simulink library "powerlib_extras"  (Simulink 6.0)
settings: Solver=ode45  SolverMode=SingleTasking  StartTime=0.0  StopTime=10.0  RelTol=1e-3
undefined symbols (not defined in the file or in its folder): Ac, Bc, Cc, Dc, Delay_discrete, dend, DiscIntNeverNeededParam, extra_sc, j, numd, test_alpha, Ts
libraries: powerlib2 x112, powerlib_extras x70, simulink_extras x25, simulink x12, powerlib_models x8
(part 7 of 9)

== system powerlib_extras/Discrete  Control Blocks/Discrete 12-Pulse HVDC Control /2nd order BP filters ==
  A : Inport  Port=1  LatchInput=off
  B : Inport  Port=2  LatchInput=off
  C : Inport  Port=3  LatchInput=off
  Discrete  2nd-Order FilterA : powerlib_extras/Discrete  Control Blocks/Discrete  2nd-Order Filter  FilterType=Bandpass  Fo=f0  Zeta=BP/2/f0  Ts=pas  Initialize=off  Vac_Init=[0.8 -25 60]  Vdc_Init=-0.4  PlotResponse=off  param1=[1 500 0.1]
  Discrete  2nd-Order FilterB : powerlib_extras/Discrete  Control Blocks/Discrete  2nd-Order Filter  FilterType=Bandpass  Fo=f0  Zeta=BP/2/f0  Ts=pas  Initialize=off  Vac_Init=[0.8 -25 60]  Vdc_Init=-0.4  PlotResponse=off  param1=[1 500 0.1]
  Discrete  2nd-Order FilterC : powerlib_extras/Discrete  Control Blocks/Discrete  2nd-Order Filter  FilterType=Bandpass  Fo=f0  Zeta=BP/2/f0  Ts=pas  Initialize=off  Vac_Init=[0.8 -25 60]  Vdc_Init=-0.4  PlotResponse=off  param1=[1 500 0.1]
  "A " : Outport
  "B " : Outport  Port=2
  "C " : Outport  Port=3
  wires:
  Discrete  2nd-Order FilterC/1 -> "C "/1
  C/1 -> Discrete  2nd-Order FilterC/1
  Discrete  2nd-Order FilterB/1 -> "B "/1
  B/1 -> Discrete  2nd-Order FilterB/1
  Discrete  2nd-Order FilterA/1 -> "A "/1
  A/1 -> Discrete  2nd-Order FilterA/1

== system powerlib_extras/Discrete  Control Blocks/Discrete 12-Pulse HVDC Control /Alpha Control ==
  alpha_max : Inport  Port=1  LatchInput=off
  alpha_min : Inport  Port=2  LatchInput=off
  forced delay : Inport  Port=3  LatchInput=off
  Data Type  Conversion : DataTypeConversion  Orientation=up  OutDataTypeMode=boolean  SaturateOnIntegerOverflow=on  RndMeth=Zero
  Data Type  Conversion1 : DataTypeConversion  OutDataTypeMode=boolean  SaturateOnIntegerOverflow=on  RndMeth=Zero
  Logical Operator : Logic  Operator=OR
  Switch : Switch  Threshold=0.5  SaturateOnIntegerOverflow=on  InputSameDT=on
  Switch1 : Switch  Threshold=0.5  SaturateOnIntegerOverflow=on  InputSameDT=on
  alpha_min_inv (deg)2 : Constant  Value=test_alpha
  fixed alpha (degrees) : Constant  Value=alpha_fix
  max_i : Outport
  min_i : Outport  Port=2
  wires:
  Data Type  Conversion1/1 -> Logical Operator/1
  alpha_min_inv (deg)2/1 -> Data Type  Conversion1/1
  Data Type  Conversion/1 -> Logical Operator/2
  forced delay/1 -> Data Type  Conversion/1
  fixed alpha (degrees)/1 -> Switch1/1, Switch/1
  Switch1/1 -> min_i/1
  Switch/1 -> max_i/1
  alpha_min/1 -> Switch1/3
  alpha_max/1 -> Switch/3
  Logical Operator/1 -> Switch1/2, Switch/2  "alpha i control"

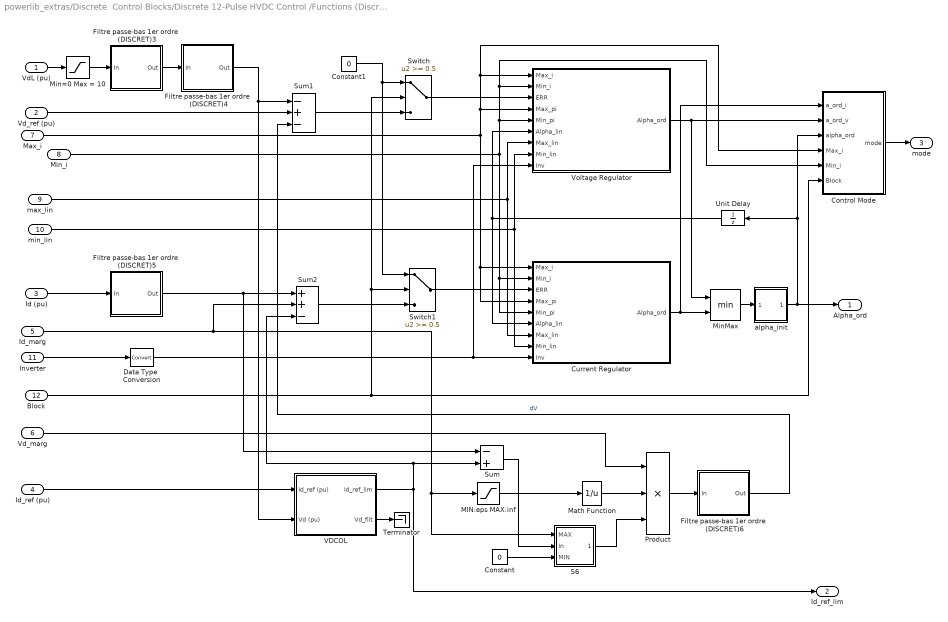
== system powerlib_extras/Discrete  Control Blocks/Discrete 12-Pulse HVDC Control /Functions (Discrete) ==
  VdL (pu) : Inport  Port=1  LatchInput=off
  Vd_ref (pu) : Inport  Port=2  LatchInput=off
  Id (pu) : Inport  Port=3  LatchInput=off
  Id_ref (pu) : Inport  Port=4  LatchInput=off
  Id_marg : Inport  Port=5  LatchInput=off
  Vd_marg : Inport  Port=6  LatchInput=off
  Max_i : Inport  Port=7  LatchInput=off
  Min_i : Inport  Port=8  LatchInput=off
  max_lin : Inport  Port=9  LatchInput=off
  min_lin : Inport  Port=10  LatchInput=off
  Inverter : Inport  Port=11  LatchInput=off
  Block : Inport  Port=12  LatchInput=off
  Constant : Constant  Value=0
  Constant1 : Constant  Value=0
  Control Mode : Subsystem
  Current Regulator : Subsystem  mask(PI Regulator  With  External  Limits (Discrete)){Kp=Kp_I, Ki=Ki_I, IC_i=ICi_I, On_lin=on, pas=pas}
      mask prompts: Kp "Kp (deg/pu):"; Ki "Ki (deg/pu/s):"; IC_i "Integrator Initial Condition (deg):"; On_lin "Linearization  (On)"; pas "Sample time (s):"
      mask help: For the linearization it is important to specifie the mode of operation i.e. rectifier or inverter (negation of rectifier).
      mask Display: disp('PI Regulator\nWith external limits\n(Linearized Kp)\n(Discrete)\n\n')
  Data Type  Conversion : DataTypeConversion  OutDataTypeMode=boolean  SaturateOnIntegerOverflow=on  RndMeth=Zero
  Filtre passe-bas 1er ordre  (DISCRET)3 : Subsystem  mask(First Order Low Pass Filter (Discrete)){T=T1_V, Pas=pas}
      mask prompts: T "Time constant T (s) :"; Pas "Time step (s)"
      mask help: H(s)=1/(1+T.s)
      mask init:
      | X=[0 1 2 3 4];
      | Y=[-2 -2 -3 -4 -4];
      | str=sprintf('\nH=1/(1+T.s)\n T= %g s\n\n\n',T);
      | num=1;
      | den=[T 1];
      | if exist('control/tf/tf')
      |    sys=tf(num,den);
      |    sysd=c2d(sys,Pas,'tustin');
      |    sys=tf(sysd);
      |    [numd,dend]=tfdata(sys,'v');
      | else
      |    [a,b,c,d]=tf2ss(num,den);
      |    nstates = size(a,1);
      |    invexp = inv(eye(nstates) - (Pas/2)*a);
      |    aout = invexp*(eye(nstates) + (Pas/2)*a);
      |    bout = invexp*b;
      |    cout = c*invexp*Pas;
      |    dout = c*invexp*b*(Pas/2) + d;
      |    [numd,dend]=ss2tf(aout,bout,cout,dout,1);
      | end
      mask Display:
      | plot(X,Y);
      | disp(str);
  Filtre passe-bas 1er ordre  (DISCRET)4 : Subsystem  mask(First Order Low Pass Filter (Discrete)){T=T2_V, Pas=pas}
      mask prompts: T "Time constant T (s) :"; Pas "Time step (s)"
      mask help: H(s)=1/(1+T.s)
      mask init: same as powerlib_extras/Discrete  Control Blocks/Discrete 12-Pulse HVDC Control /Functions (Discrete)/Filtre passe-bas 1er ordre  (DISCRET)3
      mask Display:
      | plot(X,Y);
      | disp(str);
  Filtre passe-bas 1er ordre  (DISCRET)5 : Subsystem  mask(First Order Low Pass Filter (Discrete)){T=T1_I, Pas=pas}
      mask prompts: T "Time constant T (s) :"; Pas "Time step (s)"
      mask help: H(s)=1/(1+T.s)
      mask init: same as powerlib_extras/Discrete  Control Blocks/Discrete 12-Pulse HVDC Control /Functions (Discrete)/Filtre passe-bas 1er ordre  (DISCRET)3
      mask Display:
      | plot(X,Y);
      | disp(str);
  Filtre passe-bas 1er ordre  (DISCRET)6 : Subsystem  mask(First Order Low Pass Filter (Discrete)){T=0.2, Pas=pas}
      mask prompts: T "Time constant T (s) :"; Pas "Time step (s)"
      mask help: H(s)=1/(1+T.s)
      mask init: same as powerlib_extras/Discrete  Control Blocks/Discrete 12-Pulse HVDC Control /Functions (Discrete)/Filtre passe-bas 1er ordre  (DISCRET)3
      mask Display:
      | plot(X,Y);
      | disp(str);
  MIN:eps MAX:inf : Saturate  UpperLimit=inf  LowerLimit=eps
  Math Function : Math  Operator=reciprocal  SaturateOnIntegerOverflow=on
  Min=0 Max = 10 : Saturate  UpperLimit=10  LowerLimit=0
  MinMax : MinMax  Inputs=2  SaturateOnIntegerOverflow=on  InputSameDT=on
  Product : Product  Inputs=3  SaturateOnIntegerOverflow=on  InputSameDT=on
  S6 : Subsystem
      mask Type: Limiter with External Limits
      mask Display: disp('      Limiter\n')
  Sum : Sum  Inputs=-+  SaturateOnIntegerOverflow=on  InputSameDT=on
  Sum1 : Sum  Inputs=-+-  SaturateOnIntegerOverflow=on  InputSameDT=on
  Sum2 : Sum  Inputs=++-  SaturateOnIntegerOverflow=on  InputSameDT=on
  Switch : Switch  Threshold=0.5  SaturateOnIntegerOverflow=on  InputSameDT=on
  Switch1 : Switch  Threshold=0.5  SaturateOnIntegerOverflow=on  InputSameDT=on
  Terminator : Terminator
  Unit Delay : UnitDelay  Orientation=left  SampleTime=pas
  VDCOL : Subsystem  mask(Voltage Dependent Current Order Limiter  (Discrete)){Vd_seuil=Vd_seuil, Vd_min=Vd_min, Id_min=Id_min, Id_min_abs=Id_min_abs, Tu=Tup, pas=pas}
      mask prompts: Vd_seuil "Vd seuil (pu):"; Vd_min "Vd min (pu):"; Id_min "Id min (pu):"; Id_min_abs "Id min abs (pu):"; Tu "Up Time constant (s):"; pas "Sample time (s):"
      mask Display: disp('VDCOL\n (Discrete)')
  Voltage Regulator : Subsystem  mask(PI Regulator  With  External  Limits (Discrete)){Kp=Kp_V, Ki=Ki_V, IC_i=ICi_V, On_lin=on, pas=pas}
      mask prompts: Kp "Kp (deg/pu):"; Ki "Ki (deg/pu/s):"; IC_i "Integrator Initial Condition (deg):"; On_lin "Linearization  (On)"; pas "Sample time (s):"
      mask help: For the linearization it is important to specifie the mode of operation i.e. rectifier or inverter (negation of rectifier).
      mask Display: disp('PI Regulator\nWith external limits\n(Linearized Kp)\n(Discrete)\n\n')
  alpha_init : Subsystem
  Alpha_ord : Outport
  Id_ref_lim : Outport  Port=2
  mode : Outport  Port=3
  wires:
  Id_marg/1 -> Sum2/2, S6/1(MAX), MIN:eps MAX:inf/1
  Vd_ref (pu)/1 -> Sum1/2
  Id_ref (pu)/1 -> VDCOL/1(Id_ref (pu))
  Sum/1 -> S6/2(In)
  Constant/1 -> S6/3(MIN)
  VDCOL/2(Vd_filt) -> Terminator/1
  VDCOL/1(Id_ref_lim) -> Id_ref_lim/1, Sum/2, Sum2/3
  MIN:eps MAX:inf/1 -> Math Function/1
  Filtre passe-bas 1er ordre  (DISCRET)4/1(Out) -> VDCOL/2(Vd (pu)), Sum1/1
  Filtre passe-bas 1er ordre  (DISCRET)3/1(Out) -> Filtre passe-bas 1er ordre  (DISCRET)4/1(In)
  Min=0 Max = 10/1 -> Filtre passe-bas 1er ordre  (DISCRET)3/1(In)
  VdL (pu)/1 -> Min=0 Max = 10/1
  Id (pu)/1 -> Filtre passe-bas 1er ordre  (DISCRET)5/1(In)
  Filtre passe-bas 1er ordre  (DISCRET)5/1(Out) -> Sum/1, Sum2/1
  Sum1/1 -> Switch/3
  Sum2/1 -> Switch1/3
  MinMax/1 -> alpha_init/1(In1)
  Unit Delay/1 -> Current Regulator/6(Alpha_lin), Voltage Regulator/6(Alpha_lin)
  S6/1("  ") -> Product/3
  Product/1 -> Filtre passe-bas 1er ordre  (DISCRET)6/1(In)
  Vd_marg/1 -> Product/1
  Math Function/1 -> Product/2
  alpha_init/1(Out1) -> Alpha_ord/1, Unit Delay/1, Control Mode/3(alpha_ord)
  max_lin/1 -> Voltage Regulator/7(Max_lin), Current Regulator/7(Max_lin)
  min_lin/1 -> Voltage Regulator/8(Min_lin), Current Regulator/8(Min_lin)
  Filtre passe-bas 1er ordre  (DISCRET)6/1(Out) -> Sum1/3  "dV"
  Current Regulator/1(Alpha_ord) -> MinMax/2, Control Mode/1("a_ord_i ")
  Voltage Regulator/1(Alpha_ord) -> MinMax/1, Control Mode/2(a_ord_v)
  Max_i/1 -> Current Regulator/4(Max_pi), Current Regulator/1(Max_i), Voltage Regulator/4(Max_pi), Voltage Regulator/1(Max_i), Control Mode/4(Max_i)
  Min_i/1 -> Current Regulator/5(Min_pi), Current Regulator/2(Min_i), Voltage Regulator/5(Min_pi), Voltage Regulator/2(Min_i), Control Mode/5(Min_i)
  Block/1 -> Control Mode/6(Block), Switch/2, Switch1/2
  Constant1/1 -> Switch/1, Switch1/1
  Inverter/1 -> Data Type  Conversion/1
  Data Type  Conversion/1 -> Current Regulator/9(Inv), Voltage Regulator/9(Inv)
  Switch1/1 -> Current Regulator/3(ERR)
  Switch/1 -> Voltage Regulator/3(ERR)
  Control Mode/1(mode) -> mode/1

== system powerlib_extras/Discrete  Control Blocks/Discrete 12-Pulse HVDC Control /Parameter  Selection  ==
  note: Parameters
  note: Silvano Casoria
      | Laboratoire simulation de reseaux, IREQ
  Inverter : Inport  Port=1  LatchInput=off
  Id_marg_inv (pu) : Constant  Value=Id_marg
  Id_marg_rec : Constant  Value=0
  Max_lin_inv : Constant  Value=max_lin_inv
  Max_lin_rec : Constant  Value=max_lin_rec
  Min_lin_inv : Constant  Value=min_lin_inv
  Min_lin_rec : Constant  Value=min_lin_rec
  Switch{,3..7} (6 alike) : Switch  Threshold=0.5  SaturateOnIntegerOverflow=on  InputSameDT=on
  Vd_marg_inv (pu) : Constant  Value=Vd_marg
  Vd_marg_rec : Constant  Value=0
  alpha_max_rec : Constant  Value=alpha_max_rec
  alpha_max_rec1 : Constant  Value=alpha_max_inv
  alpha_min_inv (deg) : Constant  Value=alpha_min_inv
  alpha_min_rec : Constant  Value=alpha_min_rec
  Id_marg : Outport  InitialOutput=0
  Vd_marg : Outport  Port=2  InitialOutput=0
  alpha_max : Outport  Port=3  InitialOutput=0
  alpha_min : Outport  Port=4  InitialOutput=0
  max_lin : Outport  Port=5  InitialOutput=0
  min_lin : Outport  Port=6  InitialOutput=0
  wires:
  alpha_max_rec1/1 -> Switch3/1
  alpha_max_rec/1 -> Switch3/3
  Min_lin_inv/1 -> Switch7/1
  Max_lin_inv/1 -> Switch6/1
  Max_lin_rec/1 -> Switch6/3
  Min_lin_rec/1 -> Switch7/3
  Switch7/1 -> min_lin/1
  Switch6/1 -> max_lin/1
  Switch5/1 -> Vd_marg/1
  Switch4/1 -> Id_marg/1
  Switch3/1 -> alpha_max/1
  Switch/1 -> alpha_min/1
  Inverter/1 -> Switch6/2, Switch7/2, Switch5/2, Switch4/2, Switch3/2, Switch/2
  Vd_marg_inv (pu)/1 -> Switch5/1
  Vd_marg_rec/1 -> Switch5/3
  alpha_min_rec/1 -> Switch/3
  alpha_min_inv (deg)/1 -> Switch/1
  Id_marg_rec/1 -> Switch4/3
  Id_marg_inv (pu)/1 -> Switch4/1

== system powerlib_extras/Discrete  Control Blocks/Discrete 3-phase PWM Generator/2-level Type ==
  Ust : Inport  Port=1  LatchInput=off
  wt : Inport  Port=2  LatchInput=off
  Enable : EnablePort
  Carriers Generator : Subsystem
  Gain1 : Gain  Gain=-1  SaturateOnIntegerOverflow=on
  Logical Operator : Logic  Operator=NOT
  Logical Operator1 : Logic  Operator=NOT
  Mux : Mux  Inputs=[3 3]
  Mux1 : Mux  Inputs=[3 3]
  Relational Operator : RelationalOperator  InputSameDT=on
  Relational Operator2 : RelationalOperator  Operator=<=  InputSameDT=on
  Selector1 : Selector  Elements=[1 4 2 5 3 6]  InputPortWidth=6
  Selector2 : Selector  Elements=[1 4 2 5 3 6]  InputPortWidth=6
  P1 : Outport
  P2 : Outport  Port=2
  wires:
  Selector2/1 -> P2/1
  Mux1/1 -> Selector2/1
  Logical Operator1/1 -> Mux1/2
  Relational Operator2/1 -> Logical Operator1/1, Mux1/1
  Selector1/1 -> P1/1
  Mux/1 -> Selector1/1
  Logical Operator/1 -> Mux/2
  Gain1/1 -> Relational Operator2/2
  Carriers Generator/1(C) -> Gain1/1, Relational Operator/2
  Relational Operator/1 -> Mux/1, Logical Operator/1
  wt/1 -> Carriers Generator/1(theta)
  Ust/1 -> Relational Operator2/1, Relational Operator/1

== system powerlib_extras/Discrete  Control Blocks/Discrete 3-phase PWM Generator/3-level Type ==
  Ust : Inport  Port=1  LatchInput=off
  wt : Inport  Port=2  LatchInput=off
  Enable : EnablePort
  Carriers Generator : Subsystem
  Gain1 : Gain  Gain=-1  SaturateOnIntegerOverflow=on
  Gain2 : Gain  Gain=-1  SaturateOnIntegerOverflow=on
  Relational Operator : RelationalOperator  LogicOutDataTypeMode=Specify via dialog  LogicDataType=float('double')  InputSameDT=on
  Relational Operator1 : RelationalOperator  Operator=<=  LogicOutDataTypeMode=Specify via dialog  LogicDataType=float('double')  InputSameDT=on
  Relational Operator2 : RelationalOperator  Operator=<=  LogicOutDataTypeMode=Specify via dialog  LogicDataType=float('double')  InputSameDT=on
  Relational Operator3 : RelationalOperator  LogicOutDataTypeMode=Specify via dialog  LogicDataType=float('double')  InputSameDT=on
  State-to-Pulses Decoder : Subsystem
  State-to-Pulses Decoder1 : Subsystem
  Sum2 : Sum  Inputs=|+-  SaturateOnIntegerOverflow=on  InputSameDT=on
  Sum3 : Sum  Inputs=|+-  SaturateOnIntegerOverflow=on  InputSameDT=on
  P1 : Outport
  P2 : Outport  Port=2
  wires:
  Ust/1 -> Relational Operator1/1, Relational Operator2/1, Relational Operator3/1, Relational Operator/1
  State-to-Pulses Decoder1/1(Pulses) -> P2/1
  wt/1 -> Carriers Generator/1(theta)
  State-to-Pulses Decoder/1(Pulses) -> P1/1
  Relational Operator/1 -> Sum3/1
  Relational Operator1/1 -> Sum3/2
  Carriers Generator/1(C+) -> Relational Operator/2, Gain1/1
  Carriers Generator/2(C-) -> Relational Operator1/2, Gain2/1
  Relational Operator2/1 -> Sum2/1
  Relational Operator3/1 -> Sum2/2
  Gain1/1 -> Relational Operator2/2
  Gain2/1 -> Relational Operator3/2
  Sum3/1 -> State-to-Pulses Decoder/1(State)  "State (+1,0,-1)"
  Sum2/1 -> State-to-Pulses Decoder1/1(State)  "State (+1,0,-1)"

== system powerlib_extras/Discrete  Control Blocks/Discrete 3-phase PWM Generator/Internal ==
  Constant1 : Constant  Value=[0 -2*pi/3 2*pi/3]
  Constant6 : Constant  Value=Phase
  Constant7 : Constant  Value=2*pi
  Constant8 : Constant  Value=Freq
  Constant9 : Constant  Value=m
  Product1 : Product  Inputs=3  SaturateOnIntegerOverflow=on  InputSameDT=on
  Product2 : Product  SaturateOnIntegerOverflow=on  InputSameDT=on
  Sum4 : Sum  Inputs=+++  SaturateOnIntegerOverflow=on  InputSameDT=on
  Trigonometric Function1 : Trigonometry
  deg. ->rad : Gain  Gain=pi/180  SaturateOnIntegerOverflow=on
  "t " : DigitalClock  SampleTime=Ts
  "Ust " : Outport
  wires:
  Constant7/1 -> Product1/1
  Constant8/1 -> Product1/2
  "t "/1 -> Product1/3
  Product1/1 -> Sum4/1
  Constant1/1 -> Sum4/2
  Constant6/1 -> deg. ->rad/1
  deg. ->rad/1 -> Sum4/3
  Sum4/1 -> Trigonometric Function1/1
  Trigonometric Function1/1 -> Product2/2
  Constant9/1 -> Product2/1
  Product2/1 -> "Ust "/1

== system powerlib_extras/Discrete  Control Blocks/Discrete 3-phase PWM Generator/Select 2- or 3-level ==
  Select : Inport  Port=1  PortDimensions=1  LatchInput=off
  P1 (2-L) : Inport  Port=2  PortDimensions=6  LatchInput=off
  P2 (2-L) : Inport  Port=3  PortDimensions=6  LatchInput=off
  P1 (3-L) : Inport  Port=4  PortDimensions=12  LatchInput=off
  P2 (3-L) : Inport  Port=5  PortDimensions=12  LatchInput=off
  Constant7 : Constant  Value=zeros(1,12)
  Data Type Conversion1 : DataTypeConversion  OutDataTypeMode=double  SaturateOnIntegerOverflow=on  RndMeth=Zero
  Data Type Conversion3 : DataTypeConversion  OutDataTypeMode=double  SaturateOnIntegerOverflow=on  RndMeth=Zero
  Demux : Demux  Outputs=[nPulses nPulses]
  Mux : Mux  Inputs=[6 6 12]
  Mux1 : Mux  Inputs=[12 12]
  Selector1 : Selector  Elements=SelectorElements  InputPortWidth=24
  Switch : Switch  Threshold=0.5  InputSameDT=on
  P1 : Outport
  P2 : Outport  Port=2
  wires:
  Data Type Conversion1/1 -> Mux/2
  Data Type Conversion3/1 -> Mux/1
  Mux/1 -> Switch/3
  P2 (3-L)/1 -> Mux1/2
  P1 (3-L)/1 -> Mux1/1
  Demux/2 -> P2/1
  Select/1 -> Switch/2
  Demux/1 -> P1/1
  P2 (2-L)/1 -> Data Type Conversion1/1
  P1 (2-L)/1 -> Data Type Conversion3/1
  Constant7/1 -> Mux/3
  Mux1/1 -> Switch/1
  Selector1/1 -> Demux/1
  Switch/1 -> Selector1/1

== system powerlib_extras/Discrete  Control Blocks/Discrete 3-phase PWM Generator/SubSystem ==
  note: (or B or C)
  note: (or B or C)
  note: |
      | |
      | |
      | |
      | |
      | |
      | |
      | |
      | |
      | |
      | |
      | |
      | |
      | |
      | |
      | |
      | |
      | |
      | |
      | |
      | |
      | |
      | |
      | |
      | |
      | |
      | |
      | |
  note: Pulse pattern identical to Bridge 1
  note: Bridge 2
  note: Pulses P2 -->
  note: Pulse pattern identical to Bridge 1
  note: Bridge 2
  note: Pulses P2 -->
  note: 12: Q4 (phase C)
  note: 11: Q3 (phase C)
  note: 10: Q2 (phase C)
  note: 9: Q1 (phase C )
  note: 8: Q4 (phase B)
  note: 7: Q3 (phase B)
  note: 6: Q2 (phase B)
  note: 5: Q1 (phase B )
  note: Bridge 1
  note: 4: Q4 (phase A)
  note: 3: Q3 (phase A)
  note: 2: Q2 (phase A)
  note: 1: Q1 (phase A )
  note: Pulses P1 -->
  note: 6: Q2 (phase C)
  note: Bridge 1
  note: 5: Q1 (phase C)
  note: 4: Q2 (phase B)
  note: 3: Q1 (phase B)
  note: 2: Q2 (phase A)
  note: 1: Q1 (phase A )
  note: Pulses P1 -->
  note: 3-level
  note: 2-level
  note: 0 -------------------------
  note: |
      | |
      | |
      | |
      | |
      | [Q2]
      | |
      | |
      | |
      | |
  note: |
      | |
      | |
      | |
      | |
      | [Q1]
      | |
      | |
      | |
      | |
  note: Vdc --------------------
  note: ------------ A
  note: + Vdc --------------------------
  note: - Vdc--------------------------
  note: N -----------
  note: |
      | |
      | |
      | |
      | |
      | |
      | |
      | |
      | |
      | |
      | |
  note: ---------- A
  note: ----------[D]---------
  note: ----------[D]---------
  note: |
      | |
      | [Q4]
      | |
      | |
      | |
  note: |
      | |
      | [Q3]
      | |
      | |
  note: |
      | |
      | [Q2]
      | |
      | |
  note: |
      | |
      | |
      | [Q1]
      | |
      | |

== system powerlib_extras/Discrete  Control Blocks/Discrete Gamma Measurement/Commutation Voltages ==
  note: Secondary Winding Connection
      | transfo_type : 1=Y  2=D1(lag)  3=D11(lead)
  note: Suppress
      |  zero- sequence voltages
  Uabc : Inport  Port=1  LatchInput=off
  Constant3 : Constant  Value=transfo_type
  Gain1 : Gain  Gain=1/3  SaturateOnIntegerOverflow=on
  Gain2 : Gain  Gain=sqrt(3)  SaturateOnIntegerOverflow=on
  Gain3 : Gain  Gain=sqrt(3)  SaturateOnIntegerOverflow=on
  Gain5 : Gain  Gain=-1  SaturateOnIntegerOverflow=on
  Gain6 : Gain  Gain=-1  SaturateOnIntegerOverflow=on
  Multiport Switch : MultiPortSwitch  Inputs=3  SaturateOnIntegerOverflow=on
  Mux1 : Mux  Inputs=[3 3]
  Selector : Selector  Elements=[2 3 1]  InputPortWidth=3
  Selector1 : Selector  Elements=[3 1 2]  InputPortWidth=3
  Selector2 : Selector  Elements="[1 4  2  5  3  6]"  InputPortWidth=6
  Sum2 : Sum  Inputs=1  SaturateOnIntegerOverflow=on
  Sum3 : Sum  Inputs=|+-  SaturateOnIntegerOverflow=on
  Sum5 : Sum  Inputs=|++  SaturateOnIntegerOverflow=on
  Ucom (1-6) : Outport
  wires:
  Selector/1 -> Sum5/2, Gain3/1  "-Ub -Uc -Ua"
  Gain6/1 -> Selector/1
  Gain5/1 -> Selector1/1
  Constant3/1 -> Multiport Switch/1
  Sum5/1 -> Multiport Switch/2  "Uab Ubc Uca"
  Multiport Switch/1 -> Gain5/1, Mux1/1  "Ucom 1-3-5"
  Selector1/1 -> Mux1/2  "Ucom 2-4-6"
  Mux1/1 -> Selector2/1
  Uabc/1 -> Sum3/1, Sum2/1  "Uag Ubg Ucg"
  Sum2/1 -> Gain1/1
  Gain1/1 -> Sum3/2
  Sum3/1 -> Sum5/1, Gain2/1, Gain6/1  "Ua Ub Uc"
  Selector2/1 -> Ucom (1-6)/1
  Gain2/1 -> Multiport Switch/3
  Gain3/1 -> Multiport Switch/4

== system powerlib_extras/Discrete  Control Blocks/Discrete HVDC Controller/Alpha Control ==
  Forced_alpha : Inport  Port=1  LatchInput=off
  D_alpha : Inport  Port=2  LatchInput=off
  Constant1 : Constant  Value=alpha_min
  Constant2 : Constant  Value=alpha_max
  Constant3 : Constant  Value=test_alpha
  Data Type  Conversion : DataTypeConversion  Orientation=up  OutDataTypeMode=boolean  SaturateOnIntegerOverflow=on  RndMeth=Zero
  Logical Operator : Logic  Operator=OR
  "Rate Limiter " : RateLimiter  RisingSlewLimit=PRate_fix  FallingSlewLimit=NRate_fix
  "Rate Limiter   " : RateLimiter  RisingSlewLimit=PRate_fix  FallingSlewLimit=NRate_fix
  Sum : Sum  Inputs=-+  SaturateOnIntegerOverflow=on  InputSameDT=on
  Switch : Switch  Threshold=0.5  SaturateOnIntegerOverflow=on  InputSameDT=on
  Switch1 : Switch  Threshold=0.5  SaturateOnIntegerOverflow=on  InputSameDT=on
  fixed alpha (deg) : Constant  Value=alpha_fix
  Max_i : Outport
  Min_i : Outport  Port=2
  wires:
  Data Type  Conversion/1 -> Logical Operator/2
  Forced_alpha/1 -> Data Type  Conversion/1
  fixed alpha (deg)/1 -> Switch1/1, Switch/1
  Switch1/1 -> "Rate Limiter   "/1
  Switch/1 -> "Rate Limiter "/1
  Constant1/1 -> Switch1/3
  Logical Operator/1 -> Switch1/2, Switch/2
  Constant3/1 -> Logical Operator/1
  Constant2/1 -> Sum/2
  Sum/1 -> Switch/3
  D_alpha/1 -> Sum/1
  "Rate Limiter "/1 -> Max_i/1
  "Rate Limiter   "/1 -> Min_i/1

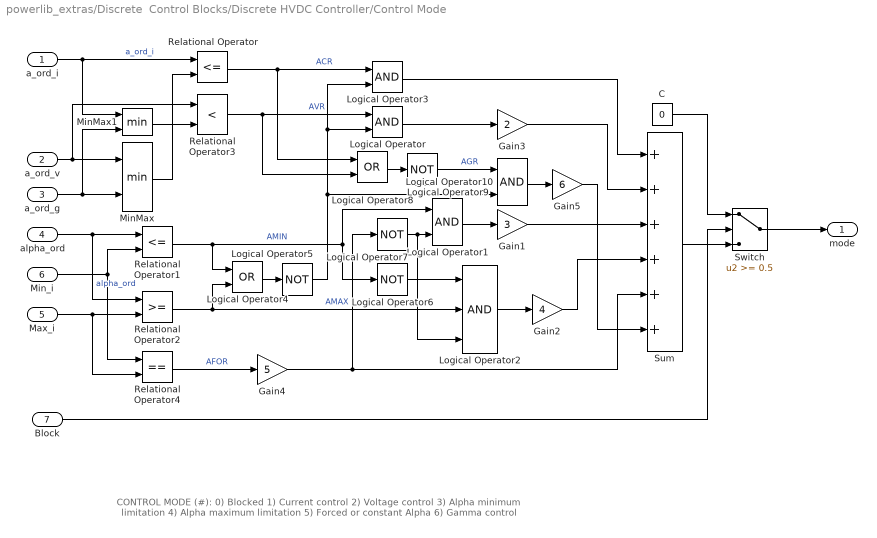
== system powerlib_extras/Discrete  Control Blocks/Discrete HVDC Controller/Control Mode  ==
  note: CONTROL MODE (#):
      |
      | 0) Blocked
      | 1) Current control
      | 2) Voltage control
      | 3) Alpha minimum limitation
      | 4) Alpha maximum limitation
      | 5) Forced or constant Alpha
      | 6) Gamma control
  "a_ord_i " : Inport  Port=1  LatchInput=off
  a_ord_v : Inport  Port=2  LatchInput=off
  a_ord_g : Inport  Port=3  LatchInput=off
  alpha_ord : Inport  Port=4  LatchInput=off
  Max_i : Inport  Port=5  LatchInput=off
  Min_i : Inport  Port=6  LatchInput=off
  Block : Inport  Port=7  LatchInput=off
  C : Constant  Value=0
  Gain1 : Gain  Gain=3  SaturateOnIntegerOverflow=on
  Gain2 : Gain  Gain=4  SaturateOnIntegerOverflow=on
  Gain3 : Gain  Gain=2  SaturateOnIntegerOverflow=on
  Gain4 : Gain  Gain=5  SaturateOnIntegerOverflow=on
  Gain5 : Gain  Gain=6  SaturateOnIntegerOverflow=on
  Logical Operator{,1,3,10} (4 alike) : Logic
  Logical Operator2 : Logic  Inputs=3
  Logical Operator4 : Logic  Operator=OR
  Logical Operator{5..7,9} (4 alike) : Logic  Operator=NOT
  Logical Operator8 : Logic  Operator=OR
  MinMax : MinMax  Inputs=2  SaturateOnIntegerOverflow=on  InputSameDT=on
  MinMax1 : MinMax  Inputs=2  SaturateOnIntegerOverflow=on  InputSameDT=on
  Relational Operator : RelationalOperator  Operator=<=  InputSameDT=on
  Relational Operator1 : RelationalOperator  Operator=<=  InputSameDT=on
  Relational Operator2 : RelationalOperator  InputSameDT=on
  Relational Operator3 : RelationalOperator  Operator=<  InputSameDT=on
  Relational Operator4 : RelationalOperator  Operator===  InputSameDT=on
  Sum : Sum  Inputs=++++++  SaturateOnIntegerOverflow=on  InputSameDT=on
  Switch : Switch  Threshold=0.5  SaturateOnIntegerOverflow=on  InputSameDT=on
  mode : Outport
  wires:
  Logical Operator10/1 -> Gain5/1
  Logical Operator9/1 -> Logical Operator10/1  "AGR"
  MinMax1/1 -> Relational Operator3/2
  Gain5/1 -> Sum/6
  Logical Operator8/1 -> Logical Operator9/1
  MinMax/1 -> Relational Operator/2
  a_ord_g/1 -> MinMax1/2, MinMax/2
  a_ord_v/1 -> Relational Operator3/1, MinMax/1
  C/1 -> Switch/1
  Sum/1 -> Switch/3
  Switch/1 -> mode/1
  Block/1 -> Switch/2
  "a_ord_i "/1 -> MinMax1/1, Relational Operator/1  "a_ord_i"
  Relational Operator/1 -> Logical Operator8/1, Logical Operator3/1  "ACR"
  Logical Operator3/1 -> Sum/1
  Gain3/1 -> Sum/2
  Relational Operator3/1 -> Logical Operator8/2, Logical Operator/1  "AVR"
  Logical Operator/1 -> Gain3/1
  alpha_ord/1 -> Relational Operator1/1, Relational Operator2/1  "alpha_ord"
  Relational Operator1/1 -> Logical Operator4/1, Logical Operator6/1, Logical Operator1/1  "AMIN"
  Logical Operator4/1 -> Logical Operator5/1
  Relational Operator2/1 -> Logical Operator4/2, Logical Operator2/2  "AMAX"
  Logical Operator6/1 -> Logical Operator2/1
  Logical Operator2/1 -> Gain2/1
  Gain1/1 -> Sum/3
  Gain2/1 -> Sum/4
  Min_i/1 -> Relational Operator1/2, Relational Operator4/1
  Max_i/1 -> Relational Operator2/2, Relational Operator4/2
  Relational Operator4/1 -> Gain4/1  "AFOR"
  Logical Operator1/1 -> Gain1/1
  Gain4/1 -> Sum/5, Logical Operator7/1
  Logical Operator7/1 -> Logical Operator1/2, Logical Operator2/3
  Logical Operator5/1 -> Logical Operator10/2, Logical Operator/2, Logical Operator3/2

== system powerlib_extras/Discrete  Control Blocks/Discrete HVDC Controller/Current Regulator ==
  note: PI Regulator With external limits (Linearized Kp) (Discrete)
  Max_i : Inport  Port=1  LatchInput=off
  Min_i : Inport  Port=2  LatchInput=off
  ERR : Inport  Port=3  LatchInput=off
  Max_pi : Inport  Port=4  LatchInput=off
  Min_pi : Inport  Port=5  LatchInput=off
  Alpha_lin : Inport  Port=6  LatchInput=off
  Max_lin : Inport  Port=7  LatchInput=off
  Min_lin : Inport  Port=8  LatchInput=off
  Inv : Inport  Port=9  LatchInput=off
  Ground : Ground
  KI (deg per pu per s) : Gain  Gain=Ki  SaturateOnIntegerOverflow=on
  Kp (deg per pu) : Constant  Value=Kp
  Kp Linearisation : Subsystem
  Prod : Product  SaturateOnIntegerOverflow=on  InputSameDT=on
  S16 : Subsystem  mask(Integrator  With  External  Dynamic  Limits (Discrete)){k=1, ic=IC_i, dt=dt}
      mask prompts: k "Gain:"; ic "Initial Condition:"; dt "Sample time: (s)"
      mask Display: disp('Integrator\nwith\nExternal Limits\nGain & Reset & Hold\n(Discrete)')
  S6 : Subsystem
      mask Type: Limiter with External Limits
      mask Display: disp('      Limiter\n')
  Sum : Sum  SaturateOnIntegerOverflow=on  InputSameDT=on
  Alpha_ord : Outport  InitialOutput=0
  wires:
  Prod/1 -> Sum/1
  Min_lin/1 -> Kp Linearisation/4(Min_lin)
  Max_lin/1 -> Kp Linearisation/5(Max_lin)
  Inv/1 -> Kp Linearisation/3(Inv)
  Ground/1 -> S16/6(Reset Value), S16/5(Hold), S16/4(Reset)
  ERR/1 -> Prod/2, KI (deg per pu per s)/1
  S16/1(Out) -> Sum/2
  Min_pi/1 -> S6/3(MIN)
  Max_pi/1 -> S6/1(MAX)
  Sum/1 -> S6/2(In)
  Min_i/1 -> S16/2(Min)
  Max_i/1 -> S16/1(Max)
  KI (deg per pu per s)/1 -> S16/3(In)
  Kp (deg per pu)/1 -> Kp Linearisation/2(Kp)
  Kp Linearisation/1(Kp_lin) -> Prod/1
  S6/1("  ") -> Alpha_ord/1
  Alpha_lin/1 -> Kp Linearisation/1(Alpha_lin)

== system powerlib_extras/Discrete  Control Blocks/Discrete HVDC Controller/Gamma Error ==
  G_ref : Inport  Port=1  LatchInput=off
  G_meas : Inport  Port=2  LatchInput=off
  Block : Inport  Port=3  LatchInput=off
  Id_err : Inport  Port=4  LatchInput=off
  Enable : EnablePort
  Constant1 : Constant  Value=0
  Constant2 : Constant  Value=0
  Constant3 : Constant  Value=G_marg
  Constant4 : Constant  Value=Id_marg
  Discrete 1st-Order Filter : powerlib_extras/Discrete  Control Blocks/Discrete 1st-Order Filter  FilterType=Highpass  Tc=0.01  Ts=dt  Initialize=off  Vac_Init=[0.8 -25 60]  Vdc_Init=-0.4  PlotResponse=off  param1=[1 500 0.1]
  MIN:eps MAX:inf : Saturate  UpperLimit=inf  LowerLimit=eps
  Math Function : Math  Operator=reciprocal  SaturateOnIntegerOverflow=on
  Product1 : Product  Inputs=3  SaturateOnIntegerOverflow=on  InputSameDT=on
  S6 : Subsystem
      mask Type: Limiter with External Limits
      mask Display: disp('      Limiter\n')
  Sum3 : Sum  Inputs=-+-  SaturateOnIntegerOverflow=on  InputSameDT=on
  Switch2 : Switch  Threshold=0.5  SaturateOnIntegerOverflow=on  InputSameDT=on
  ERR_G : Outport
  wires:
  Constant3/1 -> Product1/1
  Id_err/1 -> S6/2(In)
  Discrete 1st-Order Filter/1 -> Sum3/3  "dG"
  Product1/1 -> Discrete 1st-Order Filter/1
  Constant4/1 -> S6/1(MAX), MIN:eps MAX:inf/1
  MIN:eps MAX:inf/1 -> Math Function/1
  Math Function/1 -> Product1/2
  S6/1("  ") -> Product1/3
  Constant2/1 -> S6/3(MIN)
  Switch2/1 -> ERR_G/1  "ERR"
  Block/1 -> Switch2/2
  Constant1/1 -> Switch2/1
  G_meas/1 -> Sum3/2
  G_ref/1 -> Sum3/1
  Sum3/1 -> Switch2/3

== system powerlib_extras/Discrete  Control Blocks/Discrete HVDC Controller/Gamma Regulator ==
  Max_i : Inport  Port=1  LatchInput=off
  Min_i : Inport  Port=2  LatchInput=off
  ERR : Inport  Port=3  LatchInput=off
  Max_pi : Inport  Port=4  LatchInput=off
  Min_pi : Inport  Port=5  LatchInput=off
  Alpha_lin : Inport  Port=6  LatchInput=off
  Max_lin : Inport  Port=7  LatchInput=off
  Min_lin : Inport  Port=8  LatchInput=off
  Inv : Inport  Port=9  LatchInput=off
  Enable : EnablePort
  Gamma Regulator : Subsystem  mask(PI Regulator  With  External  Limits (Discrete)){Kp=Kp_G, Ki=Ki_G, IC_i=ICi_G, On_lin=on, pas=dt}
      mask prompts: Kp "Kp (deg/pu):"; Ki "Ki (deg/pu/s):"; IC_i "Integrator Initial Condition (deg):"; On_lin "Linearization  (On)"; pas "Sample time (s):"
      mask help: For the linearization it is important to specifie the mode of operation i.e. rectifier or inverter (negation of rectifier).
      mask Display: disp('PI Regulator\nWith external limits\n(Linearized Kp)\n(Discrete)\n\n')
  Alpha_ord : Outport
  wires:
  Inv/1 -> Gamma Regulator/9(Inv)
  Min_lin/1 -> Gamma Regulator/8(Min_lin)
  Max_lin/1 -> Gamma Regulator/7(Max_lin)
  Alpha_lin/1 -> Gamma Regulator/6(Alpha_lin)
  Min_pi/1 -> Gamma Regulator/5(Min_pi)
  Max_pi/1 -> Gamma Regulator/4(Max_pi)
  ERR/1 -> Gamma Regulator/3(ERR)
  Min_i/1 -> Gamma Regulator/2(Min_i)
  Max_i/1 -> Gamma Regulator/1(Max_i)
  Gamma Regulator/1(Alpha_ord) -> Alpha_ord/1

== system powerlib_extras/Discrete  Control Blocks/Discrete HVDC Controller/Voltage Dependant Current Order Limiter ==
  note: Voltage Dependant Current Order Limiter (VDCOL) (Discrete)
  Id_ref (pu) : Inport  Port=1  LatchInput=off
  Vd (pu) : Inport  Port=2  LatchInput=off
  Constant : Constant  Value=Id_min
  Constant1 : Constant  Value=Vd_min
  Constant2 : Constant  Value=Vd_seuil
  Constant3 : Constant
  Constant4 : Constant
  Constant5 : Constant  Value=Tu
  Logical Operator : Logic  Orientation=left  Operator=NOT
  Math Function : Math  Operator=reciprocal  SaturateOnIntegerOverflow=on
  Max = 10 Min=Id_min_abs : Saturate  UpperLimit=10  LowerLimit=Id_min_abs
  MinMax2 : MinMax  Function=max  Inputs=2  SaturateOnIntegerOverflow=on  InputSameDT=on
  MinMax3 : MinMax  Inputs=2  SaturateOnIntegerOverflow=on  InputSameDT=on
  PB_R : Subsystem  mask(Low Pass Filter With Reset (discrete: Zoh method, Forward Euler)){ic=1, dt=pas}
      mask prompts: ic "Initial condition:"; dt "Sample time (s)"
      mask help:
      | The output will be reset to the input value (Time constant = 0)  during the input (2) is True. The Time constant (T) is defined by
      | input (3).
      mask Display:
      | plot(0,0,100,100,[90,80,70,60,50,40,29,20,10],[60,55,52,55,60,65,67,65,60],[89,80,71,60,50,40,30,20,10],[40,35,32,35,40,45,47,45,40],[56,44],[70,50]);
      | disp('\n\nD')
  Product{,1..4} (5 alike) : Product  SaturateOnIntegerOverflow=on  InputSameDT=on
  Relational Operator : RelationalOperator  InputSameDT=on
  Sum : Sum  Inputs=+-  SaturateOnIntegerOverflow=on  InputSameDT=on
  Sum1 : Sum  Inputs=+-  SaturateOnIntegerOverflow=on  InputSameDT=on
  Sum2 : Sum  Inputs=+-  SaturateOnIntegerOverflow=on  InputSameDT=on
  Sum3 : Sum  SaturateOnIntegerOverflow=on  InputSameDT=on
  Unit Delay : UnitDelay  Orientation=left  SampleTime=pas
  Id_ref_lim : Outport  InitialOutput=0
  Vd_filt : Outport  Port=2  InitialOutput=0
  wires:
  Logical Operator/1 -> PB_R/2(Reset)
  Unit Delay/1 -> Logical Operator/1
  Vd (pu)/1 -> Relational Operator/1, PB_R/1("In ")
  PB_R/1(Out) -> Relational Operator/2, Vd_filt/1, Product2/2
  Constant5/1 -> PB_R/3(T)
  Constant3/1 -> Sum/1
  Constant1/1 -> Sum1/2
  Sum1/1 -> Math Function/1
  Sum/1 -> Product/1
  Math Function/1 -> Product/2
  Constant4/1 -> Sum2/1
  Sum2/1 -> Sum3/1  "B"
  Product2/1 -> Sum3/2
  Sum3/1 -> Product1/2
  Constant/1 -> Sum/2, Product4/1
  Product4/1 -> Max = 10 Min=Id_min_abs/1  "min"
  Id_ref (pu)/1 -> Product1/1, MinMax3/1, Product4/2
  MinMax3/1 -> Id_ref_lim/1
  Product3/1 -> Sum2/2
  Product/1 -> Product2/1, Product3/2  "A"
  Constant2/1 -> Sum1/1, Product3/1
  Product1/1 -> MinMax2/1  "Idref_lim"
  MinMax2/1 -> MinMax3/2
  Max = 10 Min=Id_min_abs/1 -> MinMax2/2
  Relational Operator/1 -> Unit Delay/1

== system powerlib_extras/Discrete  Control Blocks/Discrete HVDC Controller/Voltage Error ==
  Vd_ref : Inport  Port=1  LatchInput=off
  Vd_meas : Inport  Port=2  LatchInput=off
  Block : Inport  Port=3  LatchInput=off
  Id_err : Inport  Port=4  LatchInput=off
  Enable : EnablePort
  Constant1 : Constant  Value=0
  Constant2 : Constant  Value=0
  Constant3 : Constant  Value=Vd_marg
  Constant4 : Constant  Value=Id_marg
  Discrete 1st-Order Filter : powerlib_extras/Discrete  Control Blocks/Discrete 1st-Order Filter  FilterType=Highpass  Tc=0.01  Ts=dt  Initialize=off  Vac_Init=[0.8 -25 60]  Vdc_Init=-0.4  PlotResponse=off  param1=[1 500 0.1]
  MIN:eps MAX:inf : Saturate  UpperLimit=inf  LowerLimit=eps
  Math Function : Math  Operator=reciprocal  SaturateOnIntegerOverflow=on
  Product1 : Product  Inputs=3  SaturateOnIntegerOverflow=on  InputSameDT=on
  S6 : Subsystem
      mask Type: Limiter with External Limits
      mask Display: disp('      Limiter\n')
  Sum3 : Sum  Inputs=+--  SaturateOnIntegerOverflow=on  InputSameDT=on
  Switch2 : Switch  Threshold=0.5  SaturateOnIntegerOverflow=on  InputSameDT=on
  ERR_V : Outport
  wires:
  Sum3/1 -> Switch2/3
  Vd_ref/1 -> Sum3/1
  Vd_meas/1 -> Sum3/2
  Constant1/1 -> Switch2/1
  Block/1 -> Switch2/2
  Switch2/1 -> ERR_V/1  "ERR"
  Constant2/1 -> S6/3(MIN)
  S6/1("  ") -> Product1/3
  Math Function/1 -> Product1/2
  MIN:eps MAX:inf/1 -> Math Function/1
  Constant4/1 -> MIN:eps MAX:inf/1, S6/1(MAX)
  Product1/1 -> Discrete 1st-Order Filter/1
  Discrete 1st-Order Filter/1 -> Sum3/3  "dV"
  Id_err/1 -> S6/2(In)
  Constant3/1 -> Product1/1

== system powerlib_extras/Discrete  Control Blocks/Discrete HVDC Controller/Voltage Regulator ==
  Max_i : Inport  Port=1  LatchInput=off
  Min_i : Inport  Port=2  LatchInput=off
  ERR : Inport  Port=3  LatchInput=off
  Max_pi : Inport  Port=4  LatchInput=off
  Min_pi : Inport  Port=5  LatchInput=off
  Alpha_lin : Inport  Port=6  LatchInput=off
  Max_lin : Inport  Port=7  LatchInput=off
  Min_lin : Inport  Port=8  LatchInput=off
  Inv : Inport  Port=9  LatchInput=off
  Enable : EnablePort
  Voltage Regulator : Subsystem  mask(PI Regulator  With  External  Limits (Discrete)){Kp=Kp_V, Ki=Ki_V, IC_i=ICi_V, On_lin=on, pas=dt}
      mask prompts: Kp "Kp (deg/pu):"; Ki "Ki (deg/pu/s):"; IC_i "Integrator Initial Condition (deg):"; On_lin "Linearization  (On)"; pas "Sample time (s):"
      mask help: For the linearization it is important to specifie the mode of operation i.e. rectifier or inverter (negation of rectifier).
      mask Display: disp('PI Regulator\nWith external limits\n(Linearized Kp)\n(Discrete)\n\n')
  Alpha_ord : Outport
  wires:
  Voltage Regulator/1(Alpha_ord) -> Alpha_ord/1
  Max_i/1 -> Voltage Regulator/1(Max_i)
  Min_i/1 -> Voltage Regulator/2(Min_i)
  ERR/1 -> Voltage Regulator/3(ERR)
  Max_pi/1 -> Voltage Regulator/4(Max_pi)
  Min_pi/1 -> Voltage Regulator/5(Min_pi)
  Alpha_lin/1 -> Voltage Regulator/6(Alpha_lin)
  Max_lin/1 -> Voltage Regulator/7(Max_lin)
  Min_lin/1 -> Voltage Regulator/8(Min_lin)
  Inv/1 -> Voltage Regulator/9(Inv)

== system powerlib_extras/Discrete  Control Blocks/Discrete HVDC Controller/alpha_init ==
  In1 : Inport  Port=1  PortDimensions=1  LatchInput=off
  IC : InitialCondition  Value=min([ICi_V,ICi_I,ICi_G])
  Out1 : Outport
  wires:
  In1/1 -> IC/1
  IC/1 -> Out1/1

== system powerlib_extras/Discrete  Control Blocks/Discrete SV PWM Generator/Determine reference vector (U*) ==
  note: Pha_U* (rad)
      | or
      | U* beta
  note: Mag_U*
      | or
      | U* alpha
  In1 : Inport  Port=1  LatchInput=off
  In2 : Inport  Port=2  LatchInput=off
  m_Int : Inport  Port=3  LatchInput=off
  Freq_Int : Inport  Port=4  LatchInput=off
  Pha_Init : Inport  Port=5  LatchInput=off
  "0<m<1 " : Saturate  UpperLimit=1  LowerLimit=0
  Cartesian to Polar : simulink_extras/Transformations/Cartesian to Polar
  Clock : Clock
      settings: Decimation=10
  Constant : Constant  Value=3
  Constant1 : Constant
  Constant2 : Constant  Value=2*pi
  Constant3 : Constant  Value=InputType
  Deg->Rad : Gain  Gain=pi/180  SaturateOnIntegerOverflow=on
  Freq1 : Constant  Value=pi/2
  Freq2 : Constant  Value=2*pi
  Math Function2 : Math  Operator=mod  SaturateOnIntegerOverflow=on
  Product : Product  Inputs=***  SaturateOnIntegerOverflow=on  InputSameDT=on
  Relational Operator : RelationalOperator  Operator===
  Relational Operator1 : RelationalOperator  Operator===
  Sum1 : Sum  SaturateOnIntegerOverflow=on  InputSameDT=on
  Sum2 : Sum  Inputs=+-  SaturateOnIntegerOverflow=on  InputSameDT=on
  Switch{,1..3} (4 alike) : Switch  Threshold=0.5  SaturateOnIntegerOverflow=on
  m : Outport
  alpha : Outport  Port=2
  wires:
  Sum2/1 -> Math Function2/1
  Freq1/1 -> Sum2/2
  Sum1/1 -> Switch1/1
  Switch1/1 -> Sum2/1
  Math Function2/1 -> alpha/1
  Constant2/1 -> Math Function2/2
  Clock/1 -> Product/2
  Relational Operator1/1 -> Switch3/2, Switch2/2
  Switch3/1 -> Switch1/3
  Cartesian to Polar/2 -> Switch3/3
  Cartesian to Polar/1 -> Switch2/3
  Switch2/1 -> Switch/3
  Constant3/1 -> Relational Operator/1, Relational Operator1/1
  Constant1/1 -> Relational Operator1/2
  Relational Operator/1 -> Switch/2, Switch1/2
  Constant/1 -> Relational Operator/2
  m_Int/1 -> Switch/1
  In2/1 -> Switch3/1, Cartesian to Polar/2
  In1/1 -> Switch2/1, Cartesian to Polar/1
  "0<m<1 "/1 -> m/1
  Switch/1 -> "0<m<1 "/1
  Freq2/1 -> Product/3
  Freq_Int/1 -> Product/1
  Deg->Rad/1 -> Sum1/2
  Pha_Init/1 -> Deg->Rad/1
  Product/1 -> Sum1/1

== system powerlib_extras/Discrete  Control Blocks/Discrete SV PWM Generator/INFO ==
  note: Pattern #2:
      | With this pattern, identified as "Hardware-Determined" by Texas Instruments, there is always one PWM channel staying constant for the entire PWM period.
      |  So the number of switching times for this pattern is less than pattern #1. As a result, switching losses will be reduced with Pattern #2.
  note: Pattern #1:
      | With this pattern, identified as "Software-Determined" by Texas Instruments, each PWM channel switches twice per every PWM period.
  note: --------------------------------------------------------------------------------------------------------------------------------------------------------------------
  note: Reference: Application Report SPRA524
      | Space-Vector PWM with TMS320C24x Using H/W & S/W Determined Switching Patterns
      | Zhenyu Yu, Texas Instruments
  note: The objective of the SV PWM technique is to approximate the reference voltage vector (U*) instantaneously
      | by combination of the switching states corresponding to the basic space vectors.
  note: U7 = 1 1 1
  note: Q1 Q3 Q5
  note: --------------------------------------------------------
  note: Three-Phase VSC Diagram
  note: -
  note: +
  note: --------------------------------------------------------
  note: |
      | |
      | |
  note: ---Vc
  note: |
      | |
      | |
  note: |
      | |
      | |
      | |
      | |
      | |
  note: [Q6]
  note: [Q5]
  note: |
      | |
      | |
  note: ---Vb
  note: |
      | |
      | |
  note: |
      | |
      | |
      | |
      | |
      | |
  note: [Q4]
  note: [Q3]
  note: |
      | |
      | |
  note: ---Va
  note: |
      | |
      | |
  note: |
      | |
      | |
      | |
      | |
      | |
  note: [Q2]
  note: [Q1]
  note: Vdc
  note: [n] = Sector number
  note: [2]
  note: Basic Space Vectors and Switching States
  note: U4 = 0 1 1
  note: U5 = 0 0 1
  note: U6 = 1 0 1
  note: U0 = 0 0 0
  note: U3 = 0 1 0
  note: U2 = 1 1 0
  note: U1 = 1 0 0
  note: [6]
  note: [5]
  note: [4]
  note: [3]
  note: [1]
  note: 3                       2
      |       3                   2
      |         3               2
      |           3           2
      |             3       2
      |               3   2
      | 4 4 4 4 4 4 4 4 0 1 1 1 1 1 1 1 1
      |               5   6
      |             5       6
      |           5           6
      |         5               6
      |       5                   6
      |     5                       6
  note: Two symmetrical switching patterns have been implemented:

== system powerlib_extras/Discrete  Control Blocks/Discrete SV PWM Generator/SV Modulator Pattern #1 ==
  m : Inport  Port=1  LatchInput=off
  alpha : Inport  Port=2  LatchInput=off
  Enable : EnablePort
  "Compute time duration of switching states (Ta,Tb,To) " : Subsystem
  "Determine the sector of U* based on alpha (rad). Also, determine if the sector number is odd" : Subsystem
  Generate  pulse pattern : Subsystem
      mask init:
      | %Switching pattern:
      | pat1=[0 1 1 1 1 1 0;0 0 1 1 1 0 0;0 0 0 1 0 0 0];
      | pat1(:,:,2)=[0 0 1 1 1 0 0;0 1 1 1 1 1 0;0 0 0 1 0 0 0];
      | pat1(:,:,3)=[0 0 0 1 0 0 0;0 1 1 1 1 1 0;0 0 1 1 1 0 0];
      | pat1(:,:,4)=[0 0 0 1 0 0 0;0 0 1 1 1 0 0;0 1 1 1 1 1 0];
      | pat1(:,:,5)=[0 0 1 1 1 0 0;0 0 0 1 0 0 0;0 1 1 1 1 1 0];
      | pat1(:,:,6)=[0 1 1 1 1 1 0;0 0 0 1 0 0 0;0 0 1 1 1 0 0];
  INFO : Subsystem
      mask Display: disp('?')
  Pulses : Outport
  wires:
  m/1 -> "Compute time duration of switching states (Ta,Tb,To) "/2(m)
  alpha/1 -> "Compute time duration of switching states (Ta,Tb,To) "/1(alpha), "Determine the sector of U* based on alpha (rad). Also, determine if the sector number is odd"/1(alpha)
  Generate  pulse pattern/1(Pulses) -> Pulses/1
  "Compute time duration of switching states (Ta,Tb,To) "/1(Ta_Tb_To) -> Generate  pulse pattern/2(TaTbTo)
  "Determine the sector of U* based on alpha (rad). Also, determine if the sector number is odd"/2(Odd_S) -> "Compute time duration of switching states (Ta,Tb,To) "/4(Odd_S)
  "Determine the sector of U* based on alpha (rad). Also, determine if the sector number is odd"/1(Sn) -> Generate  pulse pattern/1(Sn), "Compute time duration of switching states (Ta,Tb,To) "/3(Sn)

== system powerlib_extras/Discrete  Control Blocks/Discrete SV PWM Generator/SV Modulator Pattern #2 ==
  m : Inport  Port=1  LatchInput=off
  alpha : Inport  Port=2  LatchInput=off
  Enable : EnablePort
  Constant1 : Constant
  Constant2 : Constant  Value=0
  Conv_table : Subsystem
  Logical Operator{,1..4} (5 alike) : Logic  Operator=NOT  OutDataTypeMode=Specify via dialog  LogicDataType=float('double')
  "Look-Up Table  Determine the sector of U* based on alpha (rad). " : Lookup  DialogController=Simulink.DDGSource  InputValues=[0:pi/3:5*pi/3]  OutputValues=[1:6]  SaturateOnIntegerOverflow=on
  Multiport Switch : MultiPortSwitch  Inputs=6  SaturateOnIntegerOverflow=on  InputSameDT=on
  Multiport Switch1 : MultiPortSwitch  Inputs=6  SaturateOnIntegerOverflow=on  InputSameDT=on
  Multiport Switch2 : MultiPortSwitch  Inputs=6  SaturateOnIntegerOverflow=on  InputSameDT=on
  Mux : Mux  Inputs=6
  Polar to Cartesian : simulink_extras/Transformations/Polar to Cartesian
  Relational Operator : RelationalOperator  LogicOutDataTypeMode=Specify via dialog  LogicDataType=float('double')  InputSameDT=on
  Relational Operator2 : RelationalOperator  LogicOutDataTypeMode=Specify via dialog  LogicDataType=float('double')  InputSameDT=on
  Rounding Function : Rounding
  Sum : Sum  SaturateOnIntegerOverflow=on  InputSameDT=on
  Triangle : simulink/Sources/Repeating Sequence  rep_seq_t=[0 0.5/Fc 1/Fc]  rep_seq_y=[0 1 0]
  gain : Gain  Gain=sqrt(3)/2  SaturateOnIntegerOverflow=on
  Pulses : Outport
  wires:
  "Look-Up Table  Determine the sector of U* based on alpha (rad). "/1 -> Rounding Function/1
  Rounding Function/1 -> Conv_table/3(S), Multiport Switch/1, Multiport Switch1/1, Multiport Switch2/1
  Mux/1 -> Pulses/1
  Multiport Switch2/1 -> Logical Operator4/1, Mux/5
  Multiport Switch1/1 -> Logical Operator3/1, Mux/3
  Multiport Switch/1 -> Logical Operator2/1, Mux/1
  Logical Operator4/1 -> Mux/6
  Logical Operator3/1 -> Mux/4
  Logical Operator2/1 -> Mux/2
  Conv_table/1(T1N) -> Relational Operator/2, Sum/2
  Conv_table/2(T2N) -> Sum/1
  Sum/1 -> Relational Operator2/2
  Triangle/1 -> Relational Operator2/1, Relational Operator/1
  Constant1/1 -> Multiport Switch/2, Multiport Switch1/4, Multiport Switch2/6
  Relational Operator/1 -> Logical Operator/1, Multiport Switch2/4, Multiport Switch1/2, Multiport Switch/6
  Relational Operator2/1 -> Logical Operator1/1, Multiport Switch/4, Multiport Switch2/2, Multiport Switch1/6
  Logical Operator/1 -> Multiport Switch/3, Multiport Switch1/5, Multiport Switch2/7
  Logical Operator1/1 -> Multiport Switch1/3, Multiport Switch2/5, Multiport Switch/7
  Constant2/1 -> Multiport Switch2/3, Multiport Switch/5, Multiport Switch1/7
  Polar to Cartesian/1 -> Conv_table/1(Va)  "Valpha"
  Polar to Cartesian/2 -> Conv_table/2(Vb)  "Vbeta"
  m/1 -> gain/1
  alpha/1 -> "Look-Up Table  Determine the sector of U* based on alpha (rad). "/1, Polar to Cartesian/2
  gain/1 -> Polar to Cartesian/1

== system powerlib_extras/Discrete  Control Blocks/Discrete Synchronized 12-Pulse Generator/12 Flip-Flops ==
  S : Inport  Port=1  LatchInput=off
  R : Inport  Port=2  LatchInput=off
  6 Flip-Flop : Subsystem
  6 Flip-Flop1 : Subsystem
  Demux : Demux  Outputs=2
  Demux1 : Demux  Outputs=2
  Mux : Mux  Inputs=2
  Q : Outport
  wires:
  S/1 -> Demux/1
  Demux/1 -> 6 Flip-Flop/1(S)
  Demux/2 -> 6 Flip-Flop1/1(S)
  R/1 -> Demux1/1
  Demux1/2 -> 6 Flip-Flop1/2(R)
  Demux1/1 -> 6 Flip-Flop/2(R)
  6 Flip-Flop/1(Q) -> Mux/1
  Mux/1 -> Q/1
  6 Flip-Flop1/1(Q) -> Mux/2

== system powerlib_extras/Discrete  Control Blocks/Discrete Synchronized 6-Pulse Generator/6 Flip-Flop ==
  S : Inport  Port=1  LatchInput=off
  R : Inport  Port=2  LatchInput=off
  Demux : Demux  Outputs=6
  Demux1 : Demux  Outputs=6
  Mux : Mux  Inputs=6
  S-R Flip-Flop1 : Subsystem  mask(SRFlipFlop){initial_condition=0, Ts=Ts}
      mask prompts: initial_condition "Initial condition:"; Ts "Sample time:"
      mask help: S-R Flip Flop Block
  S-R Flip-Flop2 : Subsystem  mask(SRFlipFlop){initial_condition=0, Ts=Ts}
      mask prompts: initial_condition "Initial condition:"; Ts "Sample time:"
      mask help: S-R Flip Flop Block
  S-R Flip-Flop3 : Subsystem  mask(SRFlipFlop){initial_condition=0, Ts=Ts}
      mask prompts: initial_condition "Initial condition:"; Ts "Sample time:"
      mask help: S-R Flip Flop Block
  S-R Flip-Flop4 : Subsystem  mask(SRFlipFlop){initial_condition=0, Ts=Ts}
      mask prompts: initial_condition "Initial condition:"; Ts "Sample time:"
      mask help: S-R Flip Flop Block
  S-R Flip-Flop5 : Subsystem  mask(SRFlipFlop){initial_condition=0, Ts=Ts}
      mask prompts: initial_condition "Initial condition:"; Ts "Sample time:"
      mask help: S-R Flip Flop Block
  S-R Flip-Flop6 : Subsystem  mask(SRFlipFlop){initial_condition=0, Ts=Ts}
      mask prompts: initial_condition "Initial condition:"; Ts "Sample time:"
      mask help: S-R Flip Flop Block
  Terminator{,1..5} (6 alike) : Terminator
  Q : Outport
  wires:
  Demux1/6 -> S-R Flip-Flop6/2(R)
  Demux1/5 -> S-R Flip-Flop5/2(R)
  Demux1/4 -> S-R Flip-Flop4/2(R)
  Demux1/3 -> S-R Flip-Flop3/2(R)
  Demux1/2 -> S-R Flip-Flop2/2(R)
  Demux1/1 -> S-R Flip-Flop1/2(R)
  R/1 -> Demux1/1
  Demux/5 -> S-R Flip-Flop5/1(S)
  Demux/6 -> S-R Flip-Flop6/1(S)
  S/1 -> Demux/1
  Demux/4 -> S-R Flip-Flop4/1(S)
  Demux/3 -> S-R Flip-Flop3/1(S)
  Demux/2 -> S-R Flip-Flop2/1(S)
  Demux/1 -> S-R Flip-Flop1/1(S)
  S-R Flip-Flop1/2(!Q) -> Terminator/1
  S-R Flip-Flop6/1(Q) -> Mux/6
  Mux/1 -> Q/1
  S-R Flip-Flop5/1(Q) -> Mux/5
  S-R Flip-Flop4/1(Q) -> Mux/4
  S-R Flip-Flop3/1(Q) -> Mux/3
  S-R Flip-Flop2/1(Q) -> Mux/2
  S-R Flip-Flop1/1(Q) -> Mux/1
  S-R Flip-Flop2/2(!Q) -> Terminator1/1
  S-R Flip-Flop3/2(!Q) -> Terminator2/1
  S-R Flip-Flop4/2(!Q) -> Terminator3/1
  S-R Flip-Flop5/2(!Q) -> Terminator4/1
  S-R Flip-Flop6/2(!Q) -> Terminator5/1

== system powerlib_extras/Measurements/3-Phase Sequence Analyzer/Determine if pha20 are set to zero ==
  Mag120 : Inport  Port=1  LatchInput=off
  Pha120* : Inport  Port=2  LatchInput=off
  Constant4 : Constant  Value=0
  Demux : Demux  Outputs=[1 2]
  K : Gain  Gain=0.002  SaturateOnIntegerOverflow=on
  Mux1 : Mux  Inputs=[1 2]
  Relational Operator : RelationalOperator  Operator=>  InputSameDT=on
  Selector : Selector  Elements=[2 3]  InputPortWidth=3
  Selector2 : Selector  Elements=[1]  InputPortWidth=3
  Switch : Switch  Threshold=0.5  InputSameDT=on
  Pha120 : Outport
  wires:
  K/1 -> Relational Operator/2
  Selector/1 -> Relational Operator/1
  Constant4/1 -> Switch/3
  Selector2/1 -> K/1
  Mag120/1 -> Selector2/1, Selector/1
  Pha120*/1 -> Demux/1
  Mux1/1 -> Pha120/1
  Switch/1 -> Mux1/2
  Demux/2 -> Switch/1
  Demux/1 -> Mux1/1
  Relational Operator/1 -> Switch/2

== system powerlib_extras/Measurements/3-Phase Sequence Analyzer/Neg. Seq. Computation ==
  In : Inport  Port=1  LatchInput=off
  Enable : EnablePort
  Gain1 : Gain  Gain=[1 a2 a]  SaturateOnIntegerOverflow=on
  Gain3 : Gain  Gain=1/3  SaturateOnIntegerOverflow=on
  Sum : Sum  Inputs=1  SaturateOnIntegerOverflow=on  InputSameDT=on
  Out : Outport
  wires:
  Gain1/1 -> Sum/1
  Sum/1 -> Gain3/1
  In/1 -> Gain1/1
  Gain3/1 -> Out/1
